simulink model "eCS_Algo_Simulation_2015b"  (R2015b)
settings: Solver=ode1  StartTime=0.0  StopTime=3  FixedStep=1/80000  RelTol=1e-3
PreLoadFcn:
  | if exist('tl_preloadfcn','file'), tl_preloadfcn(gcs,402); end
PostLoadFcn:
  | , if any(exist('dsrtsu_mdlpostloadfcn', 'file') == [2, 3, 6]), try dsrtsu_mdlpostloadfcn('Execute', bdroot); catch fprintf('Error in PostLoadFcn (dsrtsu_mdlpostloadfcn) for model "%s":\n %s\n', bdroot, lasterr); end, end,
  | if exist('tl_postloadfcn','file'), tl_postloadfcn(gcs,402); end
InitFcn:
  | Omegan=1.3024e+03;
  | xi=0.9; %0.48
  | K=0.1931;
  | K1=0.0198;
  | TauLocked=0.00255;
  | TauUnLocked=0.0042;
  | Kp=1/(2*K1);
  | Ki=Kp/((TauLocked+TauUnLocked)/2);
  | if exist('tlds_init','file'), tlds_init(gcs); end
StartFcn:
  | if exist('tlds_start','file'), tlds_start(gcs); end
StopFcn:
  | if exist('tlds_stop','file'), tlds_stop(gcs); end
model workspace (MAT data in the model file):
  au8PrevExecProfile = [0 0 0 0 0 0]
values from neighbouring files (symbols this model uses):
  AccSensor = 5    [Parameter_eCS_Algo.m]
  AlgoType = 0    [Parameter_eCS_Algo.m]
  Cxy = 1*0.017    (= 0.017)    [Acc_Init_SelV1.m]
  Cxz = 1*0.017    (= 0.017)    [Acc_Init_SelV1.m]
  Cyx = 1*0.017    (= 0.017)    [Acc_Init_SelV1.m]
  Cyz = 1*0.017    (= 0.017)    [Acc_Init_SelV1.m]
  Czx = 1*0.017    (= 0.017)    [Acc_Init_SelV1.m]
  Czy = 1*0.017    (= 0.017)    [Acc_Init_SelV1.m]
  Forced_Oscillation = 0    [Parameter_eCS_Algo.m]    (also in run_Rotation_sim.m = run)
  FreqTemperature = 10    [Acc_Init_SelV1.m]
  MaxSensorOffset = 0.3    [Acc_Init_SelV1.m]
  Mean_x_noise = 4e-3    (= 0.004)    [Acc_Init_SelV1.m]
  Mean_y_noise = 4e-3    (= 0.004)    [Acc_Init_SelV1.m]
  Mean_z_noise = 4e-3    (= 0.004)    [Acc_Init_SelV1.m]
  ODR = 8000    [Acc_Init_SelV1.m]
  offsetcorrection_on_off = 0    [Parameter_eCS_Algo.m]
  phi_pulse_rotation = 0    [Parameter_eCS_Algo.m]    (also in run_Rotation_sim.m = angle)
  pulsetype = 2    [Parameter_eCS_Algo.m]    (also in run_simulation.m = j; run_simulation_ActiveX.m = j)
  Range = 4    [Acc_Init_SelV1.m]
  sensitivity_optimisation = 0    [Parameter_eCS_Algo.m]
  TempBias = 0    [Acc_Init_SelV1.m]
  TemperatureAmp = 0    [Acc_Init_SelV1.m]
  Var_x_noise = 1.84e-9    (= 1.84e-09)    [Acc_Init_SelV1.m]
  Var_y_noise = 2.025e-09    [Acc_Init_SelV1.m]
  Var_z_noise = 1.374e-09    [Acc_Init_SelV1.m]
  w_x = 2*pi*F_x    (= 376.991118431)    [Acc_Init_SelV1.m]
  w_y = 2*pi*F_y    (= 376.991118431)    [Acc_Init_SelV1.m]
  w_z = 2*pi*F_z    (= 376.991118431)    [Acc_Init_SelV1.m]
  x_max_temp_drift = 0.061    [Acc_Init_SelV1.m]
  x_offset_enable = 0    [Acc_Init_SelV1.m]
  x_run_to_run_drift = 0.0    (= 0)    [Acc_Init_SelV1.m]
  x_temp_co_drift = 0.000    (= 0)    [Acc_Init_SelV1.m]
  Xi_x = 0.7    [Acc_Init_SelV1.m]
  Xi_y = 0.7    [Acc_Init_SelV1.m]
  Xi_z = 0.7    [Acc_Init_SelV1.m]
  y_max_temp_drift = 0.061    [Acc_Init_SelV1.m]
  y_offset_enable = 0    [Acc_Init_SelV1.m]
  y_run_to_run_drift = 0.0    (= 0)    [Acc_Init_SelV1.m]
  y_temp_co_drift = 0.000    (= 0)    [Acc_Init_SelV1.m]
  z_max_temp_drift = 0.13    [Acc_Init_SelV1.m]
  z_offset_enable = 0    [Acc_Init_SelV1.m]
  z_run_to_run_drift = 0.0    (= 0)    [Acc_Init_SelV1.m]
  z_temp_co_drift = 0.000    (= 0)    [Acc_Init_SelV1.m]
undefined symbols (not defined in the file or in its folder): controller_sample_rate, ddv, DiscIntNeverNeededParam, gmw_roada_x__m_s__, gmw_roada_y__m_s__, gmw_roadtime_2kHz, KSF_50_a_x, KSF_50_a_y, KSF_50_time, KSG_30_a_x, KSG_30_a_y, KSG_30_time, Meldorf_HindenburgstraAcceleration_x__m_s_2_, Meldorf_HindenburgstraAcceleration_y__m_s_2_, Meldorf_HindenburgstraAcceleration_z__m_s_2_, Meldorf_HindenburgstraTime__s_, pulse_FF27, pulse_MPDB, pulse_ODB40, pulse_ODB64, pulse_USNCAP, pulsetime_FF27, pulsetime_MPDB, pulsetime_ODB40, pulsetime_ODB64, pulsetime_USNCAP, Rauasphalt_60_a_x, Rauasphalt_60_a_y, Rauasphalt_60_time, sigbuilder_block, VW_416_2kHza_x_2kHz, VW_416_2kHza_y_2kHz, VW_416_2kHztime_2kHz
libraries: simulink x29, tllib x23, tl_autosar_lib x15, simulink_extras x7, LIB_TF_G_111 x2, LIB_TF_G_12_StepControl x2, LIB_TF_G_112 x1, dspsigops x1
(part 3 of 13)

== system eCS_Algo_Simulation_2015b/µC Signalverarbeitung und Algorithmus2/Calculate Onset >=Threshold/Calculate Onset x-Axis ==
  Acceleration [g] : Inport
  Detect Change : simulink/Logic and Bit Operations/Detect Change  vinit=0  OutDataTypeStr=boolean
  Faktor2 : SampleTimeMath  TsampMathOp=/  TsampMathImp=Offline Scaling Adjustment
  Gain : Gain  Gain=10000/100000
  Triggered Subsystem : Subsystem  TreatAsAtomicUnit=on
  delta x : Sum  Inputs=+-
  Onset [g/s] : Outport
  wires:
  Gain/1 -> Onset [g/s]/1
  Faktor2/1 -> Triggered Subsystem/1(In), Detect Change/1, delta x/1
  Detect Change/1 -> Triggered Subsystem/Trigger
  Triggered Subsystem/1(Out1) -> delta x/2
  delta x/1 -> Gain/1
  Acceleration [g]/1 -> Faktor2/1

== system eCS_Algo_Simulation_2015b/µC Signalverarbeitung und Algorithmus2/Calculate Onset >=Threshold/Calculate Onset y-Axis ==
  Acceleration [g] : Inport
  Detect Change : simulink/Logic and Bit Operations/Detect Change  vinit=0  OutDataTypeStr=boolean
  Faktor2 : SampleTimeMath  TsampMathOp=/  TsampMathImp=Offline Scaling Adjustment
  Gain : Gain  Gain=10000/100000
  Triggered Subsystem : Subsystem  TreatAsAtomicUnit=on
  delta x : Sum  Inputs=+-
  Onset [g/s] : Outport
  wires:
  Acceleration [g]/1 -> Faktor2/1
  delta x/1 -> Gain/1
  Triggered Subsystem/1(Out1) -> delta x/2
  Detect Change/1 -> Triggered Subsystem/Trigger
  Faktor2/1 -> Triggered Subsystem/1(In), delta x/1, Detect Change/1
  Gain/1 -> Onset [g/s]/1

== system eCS_Algo_Simulation_2015b/µC Signalverarbeitung und Algorithmus2/Calculate Onset >=Threshold/Calculate Onset z-Axis ==
  Acceleration [g] : Inport
  Detect Change : simulink/Logic and Bit Operations/Detect Change  vinit=0  OutDataTypeStr=boolean
  Faktor2 : SampleTimeMath  TsampMathOp=/  TsampMathImp=Offline Scaling Adjustment
  Gain : Gain  Gain=10000/100000
  Sample and Hold : dspsigops/Sample and Hold  Commented=on  trig=Rising edge  initCond=-controller_sample_rate  latchinput=on
  Triggered Subsystem : Subsystem  TreatAsAtomicUnit=on
  delta x : Sum  Inputs=+-
  Onset [g/s] : Outport
  wires:
  Gain/1 -> Onset [g/s]/1
  Faktor2/1 -> Triggered Subsystem/1(In), Detect Change/1, delta x/1
  Detect Change/1 -> Triggered Subsystem/Trigger
  Triggered Subsystem/1(Out1) -> delta x/2
  delta x/1 -> Gain/1
  Acceleration [g]/1 -> Faktor2/1

== system eCS_Algo_Simulation_2015b/FSM/Subsystem/FSM/FSM ==
  prrEcsAlgoFlag : Inport
  prrVehicleInputs : Inport  Port=2
  prrExecutedProfiles : Inport  Port=3
  prrLdoAutotestResults : Inport  Port=4
  BusSelector : BusSelector  OutputSignals=b8EcsFlag,u16BallPosition
  BusSelector1 : BusSelector  OutputSignals=u16Vx,u8BuckleState
  BusSelector2 : BusSelector  OutputSignals=u8ExecutedProfile,u8ExecutedProfileOld
  FSM_runCheckVehicleInputs : Subsystem  TreatAsAtomicUnit=on
  FSM_runMainFunction : Subsystem  TreatAsAtomicUnit=on
  PP_psrFsmProfile : tl_autosar_lib/SWC SenderPort  data={'softwarecomponent','AUTOLIV/SoftwareComponents/FSM/FSM','port','psrFsmProfile','date',738308.66468155093}  displaystring=FSM\npsrFsmProfile
  PP_psrSolenoidState : tl_autosar_lib/SWC SenderPort  data={'softwarecomponent','AUTOLIV/SoftwareComponents/FSM/FSM','port','psrSolenoidState','date',738308.6646808217}  displaystring=FSM\npsrSolenoidState
  RP_prrEcsAlgoFlag : tl_autosar_lib/SWC ReceiverPort  data={'softwarecomponent','AUTOLIV/SoftwareComponents/FSM/FSM','port','prrEcsAlgoFlag','date',738304.65103918978}  displaystring=FSM\nprrEcsAlgoFlag
  RP_prrExecutedProfiles : tl_autosar_lib/SWC ReceiverPort  data={'softwarecomponent','AUTOLIV/SoftwareComponents/FSM/FSM','port','prrExecutedProfiles','date',738314.4322294445}  displaystring=FSM\nprrExecutedProfiles
  RP_prrLdoAutotestResults : tl_autosar_lib/SWC ReceiverPort  data={'softwarecomponent','AUTOLIV/SoftwareComponents/FSM/FSM','port','prrLdoAutotestResults','date',738560.69044597226}  displaystring=FSM\nprrLdoAutotestResults
  RP_prrVehicleInputs : tl_autosar_lib/SWC ReceiverPort  data={'softwarecomponent','AUTOLIV/SoftwareComponents/FSM/FSM','port','prrVehicleInputs','date',738304.65103979164}  displaystring=FSM\nprrVehicleInputs
  Terminator{,1..3} (4 alike) : Terminator
  psrSolenoidState : Outport
  psrFsmProfile : Outport  Port=2
  pclPwmServices_SetDutyCycle : Outport  Port=3
  wires:
  prrEcsAlgoFlag/1 -> RP_prrEcsAlgoFlag/1
  RP_prrEcsAlgoFlag/1 -> BusSelector/1
  prrVehicleInputs/1 -> RP_prrVehicleInputs/1
  RP_prrVehicleInputs/1 -> BusSelector1/1
  BusSelector/1 -> FSM_runMainFunction/1(drparg_b8EcsFlag)  "<b8EcsFlag>"
  BusSelector1/1 -> FSM_runCheckVehicleInputs/1(drparg_u16Vx)  "<u16Vx>"
  BusSelector1/2 -> FSM_runCheckVehicleInputs/2(drparg_u8BuckleState)  "<u8BuckleState>"
  FSM_runCheckVehicleInputs/1(ab8IsSolenoidUsed) -> FSM_runMainFunction/2(ab8IsSolenoidUsed)  "ab8IsSolenoidUsed"
  PP_psrSolenoidState/1 -> psrSolenoidState/1
  PP_psrFsmProfile/1 -> psrFsmProfile/1
  FSM_runMainFunction/1(au8FsmState) -> PP_psrSolenoidState/1  "au8SolenoidState"
  FSM_runMainFunction/2(au8SelectedProfile) -> PP_psrFsmProfile/1  "au8SelectedProfile"
  prrExecutedProfiles/1 -> RP_prrExecutedProfiles/1
  RP_prrExecutedProfiles/1 -> BusSelector2/1
  BusSelector2/1 -> FSM_runMainFunction/3(drparg_u8ExecutedProfile)  "<u8ExecutedProfile>"
  BusSelector2/2 -> FSM_runMainFunction/4(drparg_u8ExecutedProfileOld)  "<u8ExecutedProfileOld>"
  FSM_runMainFunction/3(Buck_SetDutyCycle) -> pclPwmServices_SetDutyCycle/1  "pclPwmServices_SetDutyCycle"
  prrLdoAutotestResults/1 -> RP_prrLdoAutotestResults/1
  RP_prrLdoAutotestResults/1 -> FSM_runCheckVehicleInputs/3(drparg_stLdoTestsResults)  "stLdoTestsResults"
  FSM_runMainFunction/6(Buck2_SetDutyCycle) -> Terminator/1
  FSM_runMainFunction/4(EN_Buck) -> Terminator1/1
  BusSelector/2 -> Terminator2/1  "<u16BallPosition>"
  FSM_runMainFunction/5(EN_Buck2) -> Terminator3/1

== system eCS_Algo_Simulation_2015b/SAD/Subsystem/SAD/SAD ==
  prrFsmProfile : Inport
  sim_au16Current : Inport  Port=2
  BusCreator : BusCreator  Inputs=2
  PP_pseSolenoidPWM : tl_autosar_lib/SWC SenderPort  data={'softwarecomponent','AUTOLIV/SoftwareComponents/SAD/SAD','port','pseSolenoidPWM','date',738464.41481978004}  displaystring=SAD\npseSolenoidPWM
  PP_psrExecutedProfiles : tl_autosar_lib/SWC SenderPort  data={'softwarecomponent','AUTOLIV/SoftwareComponents/SAD/SAD','port','psrExecutedProfiles','date',738430.41689956014}  displaystring=SAD\npsrExecutedProfiles
  RP_prrFsmProfile : tl_autosar_lib/SWC ReceiverPort  data={'softwarecomponent','AUTOLIV/SoftwareComponents/SAD/SAD','port','prrFsmProfile','date',738430.41689993057}  displaystring=SAD\nprrFsmProfile
  SAD_Init : Subsystem  TreatAsAtomicUnit=on
  SAD_runMainFunction : Subsystem  TreatAsAtomicUnit=on
  SWC ReceiverPort : tl_autosar_lib/SWC ReceiverPort  data={'softwarecomponent','AUTOLIV/SoftwareComponents/SAD/SAD','port','prrSolenoidCurrent','date',738433.42499521992}  displaystring=SAD\nprrSolenoidCurrent
  SWC SenderPort : tl_autosar_lib/SWC SenderPort  data={'softwarecomponent','AUTOLIV/SoftwareComponents/SAD/SAD','port','sim_psrSolenoidPWM','date',738433.41609917826}  displaystring=SAD\nsim_psrSolenoidPWM
  Terminator : Terminator
  Terminator1 : Terminator
  psrExecutedProfiles : Outport
  sim_au16Pwm : Outport  Port=2
  pseSolenoidPWM : Outport  Port=3
  wires:
  prrFsmProfile/1 -> RP_prrFsmProfile/1
  PP_psrExecutedProfiles/1 -> psrExecutedProfiles/1
  BusCreator/1 -> PP_psrExecutedProfiles/1
  RP_prrFsmProfile/1 -> SAD_runMainFunction/1(drparg_au8SelectedProfile)  "au8SelectedProfile"
  SAD_runMainFunction/1(dsp_u8ExecutedProfile) -> BusCreator/1  "u8ExecutedProfile"
  SAD_runMainFunction/2(dsp_u8ExecutedProfileOld) -> BusCreator/2  "u8ExecutedProfileOld"
  SAD_Init/1(stProfileCfg) -> SAD_runMainFunction/2(stProfileCfg)  "stProfileCfg"
  SAD_runMainFunction/3(sim_au16Pwm) -> SWC SenderPort/1
  SWC SenderPort/1 -> sim_au16Pwm/1
  sim_au16Current/1 -> SWC ReceiverPort/1
  SWC ReceiverPort/1 -> SAD_runMainFunction/3(sim_au16Current)
  PP_pseSolenoidPWM/1 -> pseSolenoidPWM/1
  SAD_runMainFunction/4(dsp_au16Pwm) -> PP_pseSolenoidPWM/1  "au16Pwm"
  SAD_Init/2(EN_Boost_1) -> Terminator/1
  SAD_Init/3(EN_Boost_2) -> Terminator1/1

== system eCS_Algo_Simulation_2015b/eCS/Subsystem/eCS/eCS ==
  prrAccelMtrPerSecSqd : Inport
  prrEcsDiagRequest : Inport  Port=2
  prrSensitivityOpt : Inport  Port=3
  BusCreator : BusCreator  Inputs=2
  PP_psrEcsAlgoData : tl_autosar_lib/SWC SenderPort  data={'softwarecomponent','AUTOLIV/SoftwareComponents/eCS/eCS','port','psrEcsAlgoData','date',738573.71918493055}  displaystring=eCS\npsrEcsAlgoData
  RP_prrAccelMtrPerSecSqd : tl_autosar_lib/SWC ReceiverPort  data={'softwarecomponent','AUTOLIV/SoftwareComponents/eCS/eCS','port','prrAccelMtrPerSecSqd','date',738573.71918538189}  displaystring=eCS\nprrAccelMtrPerSecSqd
  RP_prrEcsDiagRequest : tl_autosar_lib/SWC ReceiverPort  data={'softwarecomponent','AUTOLIV/SoftwareComponents/eCS/eCS','port','prrEcsDiagRequest','date',738573.71918555559}  displaystring=eCS\nprrEcsDiagRequest
  SWC ReceiverPort : tl_autosar_lib/SWC ReceiverPort  data={'softwarecomponent','AUTOLIV/SoftwareComponents/eCS/eCS','port','prrSensitivityOpt','date',738576.35715353012}  displaystring=eCS\nprrSensitivityOpt
  eCS_runMainFunction : Subsystem  TreatAsAtomicUnit=on
  psrEcsAlgoData : Outport
  wires:
  prrAccelMtrPerSecSqd/1 -> RP_prrAccelMtrPerSecSqd/1
  prrEcsDiagRequest/1 -> RP_prrEcsDiagRequest/1
  PP_psrEcsAlgoData/1 -> psrEcsAlgoData/1
  BusCreator/1 -> PP_psrEcsAlgoData/1
  RP_prrAccelMtrPerSecSqd/1 -> eCS_runMainFunction/1(drparg_stAccelMtrPerSecSqd)  "stAccelMtrPerSecSqd"
  RP_prrEcsDiagRequest/1 -> eCS_runMainFunction/2(drparg_b8DiagReq)  "b8DiagReq"
  eCS_runMainFunction/1(dsp_b8EcsFlag) -> BusCreator/1  "b8EcsFlag"
  eCS_runMainFunction/2(dsp_u16BallPosition) -> BusCreator/2  "u16BallPosition"
  prrSensitivityOpt/1 -> SWC ReceiverPort/1
  SWC ReceiverPort/1 -> eCS_runMainFunction/3(drparg_b8IsSensitivityOpt)

== system eCS_Algo_Simulation_2015b/µC Signalverarbeitung und Algorithmus2/Calculate Onset >=Threshold/Calculate Onset x-Axis/Triggered Subsystem ==
  In : Inport  LatchByDelayingOutsideSignal=on
  Trigger : TriggerPort
  Out1 : Outport
  wires:
  In/1 -> Out1/1

== system eCS_Algo_Simulation_2015b/µC Signalverarbeitung und Algorithmus2/Calculate Onset >=Threshold/Calculate Onset y-Axis/Triggered Subsystem ==
  In : Inport  LatchByDelayingOutsideSignal=on
  Trigger : TriggerPort
  Out1 : Outport
  wires:
  In/1 -> Out1/1

== system eCS_Algo_Simulation_2015b/µC Signalverarbeitung und Algorithmus2/Calculate Onset >=Threshold/Calculate Onset z-Axis/Triggered Subsystem ==
  In : Inport  LatchByDelayingOutsideSignal=on
  Trigger : TriggerPort
  Out1 : Outport
  wires:
  In/1 -> Out1/1

== system eCS_Algo_Simulation_2015b/FSM/Subsystem/FSM/FSM/FSM_runCheckVehicleInputs ==
  drparg_u16Vx : Inport  PortDimensions=1  mask(TL_Inport){data={'autosar',{'useautosarcommunication',1,'senderreceiverport','prrVehicleInputs','dataelement','u16Vx'},'date',738304.70202324074}}
      settings: CopyFcn=if exist('tl_reset_reviewflag') == 2, tl_reset_reviewflag(gcbh); end  DeleteFcn=if exist('delete_tlblock','file')==2,delete_tlblock(gcbh);end  NameChangeFcn=if exist('rename_tlblock','file')==2,rename_tlblock(gcbh);end  OpenFcn=if exist('tl_open_blockdlg','file')==2,tl_open_blockdlg(gcbh);else,open_system(gcbh,'parameter');end
      mask Help: eval(['if exist(''tl_online_help'',''file'') == 2, tl_online_help(''Topic'',''TL_Inport''),else, web([''jar:file:///'',matlabroot,''/help/toolbox/simulink/help.jar!/slref/' lower(get_param(gcbh,'Blocktype')) '.html''], ''-helpbrowser''),end'])
      mask Display: plot([0.2 0.35 NaN 0.65 0.8],[0 1 NaN 0 1]);
  drparg_u8BuckleState : Inport  Port=2  PortDimensions=1  mask(TL_Inport){data={'autosar',{'useautosarcommunication',1,'senderreceiverport','prrVehicleInputs','dataelement','u8BuckleState'},'date',738304.7020236227}}
      settings: CopyFcn=if exist('tl_reset_reviewflag') == 2, tl_reset_reviewflag(gcbh); end  DeleteFcn=if exist('delete_tlblock','file')==2,delete_tlblock(gcbh);end  NameChangeFcn=if exist('rename_tlblock','file')==2,rename_tlblock(gcbh);end  OpenFcn=if exist('tl_open_blockdlg','file')==2,tl_open_blockdlg(gcbh);else,open_system(gcbh,'parameter');end
      mask Help: eval(['if exist(''tl_online_help'',''file'') == 2, tl_online_help(''Topic'',''TL_Inport''),else, web([''jar:file:///'',matlabroot,''/help/toolbox/simulink/help.jar!/slref/' lower(get_param(gcbh,'Blocktype')) '.html''], ''-helpbrowser''),end'])
      mask Display: plot([0.2 0.35 NaN 0.65 0.8],[0 1 NaN 0 1]);
  drparg_stLdoTestsResults : Inport  Port=3  mask(TL_BusInport){data={'#autoscaling',5,'#message',5,'#output',5,'#logdata',5,'signals',{{'stLdoTestsResults',{'u8OpenLoadResults';'u8ShortCircuitResults';'u8OverCurrentResults';'u8ThermalShutdownResults';'u8ShortToBatteryResults'}}},'autosar',{'useautosarcommunication',1,'senderreceiverport','prrLdoAutotestResults','dataelement','stLdoTestsResults'},'date',738560.69385527773}}
      settings: CopyFcn=if exist('tl_reset_reviewflag') == 2, tl_reset_reviewflag(gcbh); end  DeleteFcn=if exist('delete_tlblock','file')==2,delete_tlblock(gcbh);end  NameChangeFcn=if exist('rename_tlblock','file')==2,rename_tlblock(gcbh);end  OpenFcn=if exist('tl_open_blockdlg','file')==2,tl_open_blockdlg(gcbh);else,open_system(gcbh,'parameter');end
      mask Help: eval(['if exist(''tl_online_help'',''file'') == 2, tl_online_help(''Topic'',''TL_Inport''),else, web([''jar:file:///'',matlabroot,''/help/toolbox/simulink/help.jar!/slref/' lower(get_param(gcbh,'Blocktype')) '.html''], ''-helpbrowser''),end'])
      mask Display: plot([0.2 0.35 NaN 0.65 0.8],[0 1 NaN 0 1]);
  For Iterator Subsystem : Subsystem  TreatAsAtomicUnit=on
  Runnable : tllib/Function  data={'autosar',{'useautosarspecification',1,'softwarecomponent','AUTOLIV/SoftwareComponents/FSM/FSM','runnable','FSM_runCheckVehicleInputs'},'date',738304.7020226157}  displayString=RUNNABLE
  ab8IsSolenoidUsed : Outport  PortDimensions=6  mask(TL_Outport){data={'autosar',{'useautosarcommunication',1,'kind',3,'interrunnablevariable','ab8IsSolenoidUsed'},'date',738373.3646115741}}
      settings: CopyFcn=if exist('tl_reset_reviewflag') == 2, tl_reset_reviewflag(gcbh); end  DeleteFcn=if exist('delete_tlblock','file')==2,delete_tlblock(gcbh);end  NameChangeFcn=if exist('rename_tlblock','file')==2,rename_tlblock(gcbh);end  OpenFcn=if exist('tl_open_blockdlg','file')==2,tl_open_blockdlg(gcbh);else,open_system(gcbh,'parameter');end
      mask Help: eval(['if exist(''tl_online_help'',''file'') == 2, tl_online_help(''Topic'',''TL_Outport''),else, web([''jar:file:///'',matlabroot,''/help/toolbox/simulink/help.jar!/slref/' lower(get_param(gcbh,'Blocktype')) '.html''], ''-helpbrowser''),end'])
      mask Display: plot([0.2 0.35 NaN 0.65 0.8],[0 1 NaN 0 1]);
  wires:
  drparg_u16Vx/1 -> For Iterator Subsystem/1(u16Vx)
  drparg_u8BuckleState/1 -> For Iterator Subsystem/2(u8BuckleState)
  For Iterator Subsystem/1(ab8SolenoidEnable) -> ab8IsSolenoidUsed/1
  drparg_stLdoTestsResults/1 -> For Iterator Subsystem/3(stLdoTestResult)

== system eCS_Algo_Simulation_2015b/FSM/Subsystem/FSM/FSM/FSM_runMainFunction ==
  note: u8Level
  note: Buck PWM management
  drparg_b8EcsFlag : Inport  PortDimensions=1  mask(TL_Inport){data={'autosar',{'useautosarcommunication',1,'senderreceiverport','prrEcsAlgoFlag','dataelement','b8EcsFlag'},'date',738304.65103487263}}
      settings: CopyFcn=if exist('tl_reset_reviewflag') == 2, tl_reset_reviewflag(gcbh); end  DeleteFcn=if exist('delete_tlblock','file')==2,delete_tlblock(gcbh);end  NameChangeFcn=if exist('rename_tlblock','file')==2,rename_tlblock(gcbh);end  OpenFcn=if exist('tl_open_blockdlg','file')==2,tl_open_blockdlg(gcbh);else,open_system(gcbh,'parameter');end
      mask Help: eval(['if exist(''tl_online_help'',''file'') == 2, tl_online_help(''Topic'',''TL_Inport''),else, web([''jar:file:///'',matlabroot,''/help/toolbox/simulink/help.jar!/slref/' lower(get_param(gcbh,'Blocktype')) '.html''], ''-helpbrowser''),end'])
      mask Display: plot([0.2 0.35 NaN 0.65 0.8],[0 1 NaN 0 1]);
  ab8IsSolenoidUsed : Inport  Port=2  PortDimensions=6  mask(TL_Inport){data={'autosar',{'useautosarcommunication',1,'kind',3,'interrunnablevariable','ab8IsSolenoidUsed'},'date',738307.71878736117}}
      settings: CopyFcn=if exist('tl_reset_reviewflag') == 2, tl_reset_reviewflag(gcbh); end  DeleteFcn=if exist('delete_tlblock','file')==2,delete_tlblock(gcbh);end  NameChangeFcn=if exist('rename_tlblock','file')==2,rename_tlblock(gcbh);end  OpenFcn=if exist('tl_open_blockdlg','file')==2,tl_open_blockdlg(gcbh);else,open_system(gcbh,'parameter');end
      mask Help: eval(['if exist(''tl_online_help'',''file'') == 2, tl_online_help(''Topic'',''TL_Inport''),else, web([''jar:file:///'',matlabroot,''/help/toolbox/simulink/help.jar!/slref/' lower(get_param(gcbh,'Blocktype')) '.html''], ''-helpbrowser''),end'])
      mask Display: plot([0.2 0.35 NaN 0.65 0.8],[0 1 NaN 0 1]);
  drparg_u8ExecutedProfile : Inport  Port=3  PortDimensions=6  mask(TL_Inport){data={'logdata',{'loggingmode',1},'autosar',{'useautosarcommunication',1,'senderreceiverport','prrExecutedProfiles','dataelement','u8ExecutedProfile'},'date',738566.73895473382}}
      settings: CopyFcn=if exist('tl_reset_reviewflag') == 2, tl_reset_reviewflag(gcbh); end  DeleteFcn=if exist('delete_tlblock','file')==2,delete_tlblock(gcbh);end  NameChangeFcn=if exist('rename_tlblock','file')==2,rename_tlblock(gcbh);end  OpenFcn=if exist('tl_open_blockdlg','file')==2,tl_open_blockdlg(gcbh);else,open_system(gcbh,'parameter');end
      mask Help: eval(['if exist(''tl_online_help'',''file'') == 2, tl_online_help(''Topic'',''TL_Inport''),else, web([''jar:file:///'',matlabroot,''/help/toolbox/simulink/help.jar!/slref/' lower(get_param(gcbh,'Blocktype')) '.html''], ''-helpbrowser''),end'])
      mask Display: plot([0.2 0.35 NaN 0.65 0.8],[0 1 NaN 0 1]);
  drparg_u8ExecutedProfileOld : Inport  Port=4  PortDimensions=6  mask(TL_Inport){data={'autosar',{'useautosarcommunication',1,'senderreceiverport','prrExecutedProfiles','dataelement','u8ExecutedProfileOld'},'date',738344.68584724539}}
      settings: CopyFcn=if exist('tl_reset_reviewflag') == 2, tl_reset_reviewflag(gcbh); end  DeleteFcn=if exist('delete_tlblock','file')==2,delete_tlblock(gcbh);end  NameChangeFcn=if exist('rename_tlblock','file')==2,rename_tlblock(gcbh);end  OpenFcn=if exist('tl_open_blockdlg','file')==2,tl_open_blockdlg(gcbh);else,open_system(gcbh,'parameter');end
      mask Help: eval(['if exist(''tl_online_help'',''file'') == 2, tl_online_help(''Topic'',''TL_Inport''),else, web([''jar:file:///'',matlabroot,''/help/toolbox/simulink/help.jar!/slref/' lower(get_param(gcbh,'Blocktype')) '.html''], ''-helpbrowser''),end'])
      mask Display: plot([0.2 0.35 NaN 0.65 0.8],[0 1 NaN 0 1]);
  Bitwise Operator : tllib/Bitwise Operator  logicop=AND  UseBitMask=on  BitMask=bin2dec('00000111')  BitMaskRealWorld=Stored Integer  data={'logdata',{'loggingmode',1},'date',738566.66057049774}
  Buck PWM LuT : Lookup_n-D  NumberOfTableDimensions=1  BreakpointsForDimension1=ddv('FSM/NVP/CFG_au16TempInDeg')  BreakpointsForDimension2=[1:3]  IndexSearchMethod=Linear search  Table=ddv('FSM/NVP/CFG_au16BuckPwm')  ExtrapMethod=Clip  InternalRulePriority=Speed  RndMeth=Simplest  InputSameDT=on  mask(TL_Lookup1D){data={'input',{'variable','FSM/NVP/CFG_au16TempInDeg'},'output',{'type','UInt16'},'table',{'variable','FSM/NVP/CFG_au16BuckPwm'},'date',738597.41315780091}}
      settings: CopyFcn=if exist('tl_reset_reviewflag') == 2, tl_reset_reviewflag(gcbh); end  DeleteFcn=if exist('delete_tlblock','file')==2,delete_tlblock(gcbh);end  NameChangeFcn=if exist('rename_tlblock','file')==2,rename_tlblock(gcbh);end  OpenFcn=if exist('tl_open_blockdlg','file')==2,tl_open_blockdlg(gcbh);else,open_system(gcbh,'parameter');end
      mask Help: eval(['if exist(''tl_online_help'',''file'') == 2, tl_online_help(''Topic'',''TL_Lookup1D''),else, web([''jar:file:///'',matlabroot,''/help/toolbox/simulink/help.jar!/slref/' lower(get_param(gcbh,'Blocktype')) '.html''], ''-helpbrowser''),end'])
      mask Display: plot([-0.1, 1.05, NaN, -0.1, 1.05],[.01, .01, NaN, .99, .99]);
  BusCreator{,1..3} (4 alike) : BusCreator  Inputs=2
  Const : Constant  Value=ddv('PWMIF/Macros/Channels/PWMIF_CH_BUCK_1')  mask(TL_Constant){data={'output',{'variable','PWMIF/Macros/Channels/PWMIF_CH_BUCK_1'},'date',738597.35914218752}}
      settings: CopyFcn=if exist('tl_reset_reviewflag') == 2, tl_reset_reviewflag(gcbh); end  DeleteFcn=if exist('delete_tlblock','file')==2,delete_tlblock(gcbh);end  NameChangeFcn=if exist('rename_tlblock','file')==2,rename_tlblock(gcbh);end  OpenFcn=if exist('tl_open_blockdlg','file')==2,tl_open_blockdlg(gcbh);else,open_system(gcbh,'parameter');end
      mask Help: eval(['if exist(''tl_online_help'',''file'') == 2, tl_online_help(''Topic'',''TL_Constant''),else, web([''jar:file:///'',matlabroot,''/help/toolbox/simulink/help.jar!/slref/' lower(get_param(gcbh,'Blocktype')) '.html''], ''-helpbrowser''),end'])
      mask Display: plot([-0.1, 1.05, NaN, -0.1, 1.05],[.01, .01, NaN, .99, .99]);
  Const1 : Constant  Value=1966  mask(TL_Constant){data={'date',738478.39187206014}}
      settings: CopyFcn=if exist('tl_reset_reviewflag') == 2, tl_reset_reviewflag(gcbh); end  DeleteFcn=if exist('delete_tlblock','file')==2,delete_tlblock(gcbh);end  NameChangeFcn=if exist('rename_tlblock','file')==2,rename_tlblock(gcbh);end  OpenFcn=if exist('tl_open_blockdlg','file')==2,tl_open_blockdlg(gcbh);else,open_system(gcbh,'parameter');end
      mask Help: eval(['if exist(''tl_online_help'',''file'') == 2, tl_online_help(''Topic'',''TL_Constant''),else, web([''jar:file:///'',matlabroot,''/help/toolbox/simulink/help.jar!/slref/' lower(get_param(gcbh,'Blocktype')) '.html''], ''-helpbrowser''),end'])
      mask Display: plot([-0.1, 1.05, NaN, -0.1, 1.05],[.01, .01, NaN, .99, .99]);
  Const3 : Constant  Value=32768  mask(TL_Constant){data={'date',738478.39617783565}}
      settings: CopyFcn=if exist('tl_reset_reviewflag') == 2, tl_reset_reviewflag(gcbh); end  DeleteFcn=if exist('delete_tlblock','file')==2,delete_tlblock(gcbh);end  NameChangeFcn=if exist('rename_tlblock','file')==2,rename_tlblock(gcbh);end  OpenFcn=if exist('tl_open_blockdlg','file')==2,tl_open_blockdlg(gcbh);else,open_system(gcbh,'parameter');end
      mask Help: eval(['if exist(''tl_online_help'',''file'') == 2, tl_online_help(''Topic'',''TL_Constant''),else, web([''jar:file:///'',matlabroot,''/help/toolbox/simulink/help.jar!/slref/' lower(get_param(gcbh,'Blocktype')) '.html''], ''-helpbrowser''),end'])
      mask Display: plot([-0.1, 1.05, NaN, -0.1, 1.05],[.01, .01, NaN, .99, .99]);
  Const4 : Constant  Value=ddv('DIOIF/Macros/Channels/DIOIF_CH_EN_BUCK_1')  mask(TL_Constant){data={'output',{'variable','DIOIF/Macros/Channels/DIOIF_CH_EN_BUCK_1'},'date',738597.35860167828}}
      settings: CopyFcn=if exist('tl_reset_reviewflag') == 2, tl_reset_reviewflag(gcbh); end  DeleteFcn=if exist('delete_tlblock','file')==2,delete_tlblock(gcbh);end  NameChangeFcn=if exist('rename_tlblock','file')==2,rename_tlblock(gcbh);end  OpenFcn=if exist('tl_open_blockdlg','file')==2,tl_open_blockdlg(gcbh);else,open_system(gcbh,'parameter');end
      mask Help: eval(['if exist(''tl_online_help'',''file'') == 2, tl_online_help(''Topic'',''TL_Constant''),else, web([''jar:file:///'',matlabroot,''/help/toolbox/simulink/help.jar!/slref/' lower(get_param(gcbh,'Blocktype')) '.html''], ''-helpbrowser''),end'])
      mask Display: plot([-0.1, 1.05, NaN, -0.1, 1.05],[.01, .01, NaN, .99, .99]);
  Const5 : Constant  Value=ddv('DIOIF/Macros/Channels/DIOIF_CH_EN_BUCK_2')  mask(TL_Constant){data={'output',{'variable','DIOIF/Macros/Channels/DIOIF_CH_EN_BUCK_2'},'date',738597.358925162}}
      settings: CopyFcn=if exist('tl_reset_reviewflag') == 2, tl_reset_reviewflag(gcbh); end  DeleteFcn=if exist('delete_tlblock','file')==2,delete_tlblock(gcbh);end  NameChangeFcn=if exist('rename_tlblock','file')==2,rename_tlblock(gcbh);end  OpenFcn=if exist('tl_open_blockdlg','file')==2,tl_open_blockdlg(gcbh);else,open_system(gcbh,'parameter');end
      mask Help: eval(['if exist(''tl_online_help'',''file'') == 2, tl_online_help(''Topic'',''TL_Constant''),else, web([''jar:file:///'',matlabroot,''/help/toolbox/simulink/help.jar!/slref/' lower(get_param(gcbh,'Blocktype')) '.html''], ''-helpbrowser''),end'])
      mask Display: plot([-0.1, 1.05, NaN, -0.1, 1.05],[.01, .01, NaN, .99, .99]);
  Const6 : Constant  Value=ddv('STD_LOW')  mask(TL_Constant){data={'output',{'variable','STD_LOW'},'date',738566.49000547454}}
      settings: CopyFcn=if exist('tl_reset_reviewflag') == 2, tl_reset_reviewflag(gcbh); end  DeleteFcn=if exist('delete_tlblock','file')==2,delete_tlblock(gcbh);end  NameChangeFcn=if exist('rename_tlblock','file')==2,rename_tlblock(gcbh);end  OpenFcn=if exist('tl_open_blockdlg','file')==2,tl_open_blockdlg(gcbh);else,open_system(gcbh,'parameter');end
      mask Help: eval(['if exist(''tl_online_help'',''file'') == 2, tl_online_help(''Topic'',''TL_Constant''),else, web([''jar:file:///'',matlabroot,''/help/toolbox/simulink/help.jar!/slref/' lower(get_param(gcbh,'Blocktype')) '.html''], ''-helpbrowser''),end'])
      mask Display: plot([-0.1, 1.05, NaN, -0.1, 1.05],[.01, .01, NaN, .99, .99]);
  Const7 : Constant  Value=ddv('DIOIF/Macros/IO_Level/DIOIF_STD_HIGH')  mask(TL_Constant){data={'output',{'variable','DIOIF/Macros/IO_Level/DIOIF_STD_HIGH'},'date',738566.68557425926}}
      settings: CopyFcn=if exist('tl_reset_reviewflag') == 2, tl_reset_reviewflag(gcbh); end  DeleteFcn=if exist('delete_tlblock','file')==2,delete_tlblock(gcbh);end  NameChangeFcn=if exist('rename_tlblock','file')==2,rename_tlblock(gcbh);end  OpenFcn=if exist('tl_open_blockdlg','file')==2,tl_open_blockdlg(gcbh);else,open_system(gcbh,'parameter');end
      mask Help: eval(['if exist(''tl_online_help'',''file'') == 2, tl_online_help(''Topic'',''TL_Constant''),else, web([''jar:file:///'',matlabroot,''/help/toolbox/simulink/help.jar!/slref/' lower(get_param(gcbh,'Blocktype')) '.html''], ''-helpbrowser''),end'])
      mask Display: plot([-0.1, 1.05, NaN, -0.1, 1.05],[.01, .01, NaN, .99, .99]);
  Const8 : Constant  Value=ddv('PWMIF/Macros/Channels/PWMIF_CH_BUCK_2')  mask(TL_Constant){data={'output',{'variable','PWMIF/Macros/Channels/PWMIF_CH_BUCK_2'},'date',738597.35934738431}}
      settings: CopyFcn=if exist('tl_reset_reviewflag') == 2, tl_reset_reviewflag(gcbh); end  DeleteFcn=if exist('delete_tlblock','file')==2,delete_tlblock(gcbh);end  NameChangeFcn=if exist('rename_tlblock','file')==2,rename_tlblock(gcbh);end  OpenFcn=if exist('tl_open_blockdlg','file')==2,tl_open_blockdlg(gcbh);else,open_system(gcbh,'parameter');end
      mask Help: eval(['if exist(''tl_online_help'',''file'') == 2, tl_online_help(''Topic'',''TL_Constant''),else, web([''jar:file:///'',matlabroot,''/help/toolbox/simulink/help.jar!/slref/' lower(get_param(gcbh,'Blocktype')) '.html''], ''-helpbrowser''),end'])
      mask Display: plot([-0.1, 1.05, NaN, -0.1, 1.05],[.01, .01, NaN, .99, .99]);
  Determine Transition : Subsystem  TreatAsAtomicUnit=on
  ExecuteState : Subsystem  TreatAsAtomicUnit=on
  Multiport Switch : MultiPortSwitch  DataPortOrder=Specify indices  Inputs=6  DataPortIndices={1,2,4}  DataPortForDefault=Additional data port  DiagnosticForDefault=None  mask(TL_MultiPortSwitch){data={'output',{'type','UInt16'},'date',738589.71235600696}}
      settings: CopyFcn=if exist('tl_reset_reviewflag') == 2, tl_reset_reviewflag(gcbh); end  DeleteFcn=if exist('delete_tlblock','file')==2,delete_tlblock(gcbh);end  NameChangeFcn=if exist('rename_tlblock','file')==2,rename_tlblock(gcbh);end  OpenFcn=if exist('tl_open_blockdlg','file')==2,tl_open_blockdlg(gcbh);else,open_system(gcbh,'parameter');end
      mask Help: eval(['if exist(''tl_online_help'',''file'') == 2, tl_online_help(''Topic'',''TL_MultiPortSwitch''),else, web([''jar:file:///'',matlabroot,''/help/toolbox/simulink/help.jar!/slref/' lower(get_param(gcbh,'Blocktype')) '.html''], ''-helpbrowser''),end'])
      mask Display: plot([-0.1, 1.05, NaN, -0.1, 1.05],[.01, .01, NaN, .99, .99]);
  Runnable : tllib/Function  data={'autosar',{'useautosarspecification',1,'softwarecomponent','AUTOLIV/SoftwareComponents/FSM/FSM','runnable','FSM_runMainFunction'},'date',738304.65103259264}  displayString=RUNNABLE
  Src : Subsystem
  Switch : Switch  Criteria=u2 ~= 0  mask(TL_Switch){data={'output',{'type','AUTOLIV/DioIf_DataDictionnary/ImplementationDataTypes/u8DioIfLvlType'},'date',738566.48839523143}}
      settings: CopyFcn=if exist('tl_reset_reviewflag') == 2, tl_reset_reviewflag(gcbh); end  DeleteFcn=if exist('delete_tlblock','file')==2,delete_tlblock(gcbh);end  NameChangeFcn=if exist('rename_tlblock','file')==2,rename_tlblock(gcbh);end  OpenFcn=if exist('tl_open_blockdlg','file')==2,tl_open_blockdlg(gcbh);else,open_system(gcbh,'parameter');end
      mask Help: eval(['if exist(''tl_online_help'',''file'') == 2, tl_online_help(''Topic'',''TL_Switch''),else, web([''jar:file:///'',matlabroot,''/help/toolbox/simulink/help.jar!/slref/' lower(get_param(gcbh,'Blocktype')) '.html''], ''-helpbrowser''),end'])
      mask Display: plot([-0.1, 1.05, NaN, -0.1, 1.05],[.01, .01, NaN, .99, .99]);
  old state : UnitDelay  InitialCondition=ddv('FSM/astFsm/Components/au8FsmStatesOld')  SampleTime=-1  mask(TL_UnitDelay){data={'output',{'name','$D','inheritscaling',1},'state',{'variable','FSM/astFsm/Components/au8FsmStatesOld'},'date',738331.66886591434}}
      settings: CopyFcn=if exist('tl_reset_reviewflag') == 2, tl_reset_reviewflag(gcbh); end  DeleteFcn=if exist('delete_tlblock','file')==2,delete_tlblock(gcbh);end  NameChangeFcn=if exist('rename_tlblock','file')==2,rename_tlblock(gcbh);end  OpenFcn=if exist('tl_open_blockdlg','file')==2,tl_open_blockdlg(gcbh);else,open_system(gcbh,'parameter');end
      mask Help: eval(['if exist(''tl_online_help'',''file'') == 2, tl_online_help(''Topic'',''TL_UnitDelay''),else, web([''jar:file:///'',matlabroot,''/help/toolbox/simulink/help.jar!/slref/' lower(get_param(gcbh,'Blocktype')) '.html''], ''-helpbrowser''),end'])
      mask Display: plot([-0.1, 1.05, NaN, -0.1, 1.05],[.01, .01, NaN, .99, .99]);
  scp_getMeasure : Subsystem  TreatAsAtomicUnit=on
  au8FsmState : Outport  PortDimensions=6  mask(TL_Outport){data={'logdata',{'loggingmode',1},'autosar',{'useautosarcommunication',1,'senderreceiverport','psrSolenoidState','dataelement','au8SolenoidState'},'date',738314.63122943288}}
      settings: CopyFcn=if exist('tl_reset_reviewflag') == 2, tl_reset_reviewflag(gcbh); end  DeleteFcn=if exist('delete_tlblock','file')==2,delete_tlblock(gcbh);end  NameChangeFcn=if exist('rename_tlblock','file')==2,rename_tlblock(gcbh);end  OpenFcn=if exist('tl_open_blockdlg','file')==2,tl_open_blockdlg(gcbh);else,open_system(gcbh,'parameter');end
      mask Help: eval(['if exist(''tl_online_help'',''file'') == 2, tl_online_help(''Topic'',''TL_Outport''),else, web([''jar:file:///'',matlabroot,''/help/toolbox/simulink/help.jar!/slref/' lower(get_param(gcbh,'Blocktype')) '.html''], ''-helpbrowser''),end'])
      mask Display: plot([0.2 0.35 NaN 0.65 0.8],[0 1 NaN 0 1]);
  au8SelectedProfile : Outport  Port=2  PortDimensions=6  mask(TL_Outport){data={'logdata',{'loggingmode',1},'autosar',{'useautosarcommunication',1,'senderreceiverport','psrFsmProfile','dataelement','au8SelectedProfile'},'date',738314.63131238427}}
      settings: CopyFcn=if exist('tl_reset_reviewflag') == 2, tl_reset_reviewflag(gcbh); end  DeleteFcn=if exist('delete_tlblock','file')==2,delete_tlblock(gcbh);end  NameChangeFcn=if exist('rename_tlblock','file')==2,rename_tlblock(gcbh);end  OpenFcn=if exist('tl_open_blockdlg','file')==2,tl_open_blockdlg(gcbh);else,open_system(gcbh,'parameter');end
      mask Help: eval(['if exist(''tl_online_help'',''file'') == 2, tl_online_help(''Topic'',''TL_Outport''),else, web([''jar:file:///'',matlabroot,''/help/toolbox/simulink/help.jar!/slref/' lower(get_param(gcbh,'Blocktype')) '.html''], ''-helpbrowser''),end'])
      mask Display: plot([0.2 0.35 NaN 0.65 0.8],[0 1 NaN 0 1]);
  Buck_SetDutyCycle : Outport  Port=3  mask(TL_BusOutport){data={'#autoscaling',2,'#message',2,'#output',2,'#logdata',2,'logdata#2',{'loggingmode',1},'signals',{{'SetDutyCycle',{'cu8ChannelID';'cu16DutyCycle'}}},'autosar',{'useautosarcommunication',1,'kind',4,'clientserverport','pclPwmServices','operation','SetDutyCycle'},'date',738478.39676596061}}
      settings: CopyFcn=if exist('tl_reset_reviewflag') == 2, tl_reset_reviewflag(gcbh); end  DeleteFcn=if exist('delete_tlblock','file')==2,delete_tlblock(gcbh);end  NameChangeFcn=if exist('rename_tlblock','file')==2,rename_tlblock(gcbh);end  OpenFcn=if exist('tl_open_blockdlg','file')==2,tl_open_blockdlg(gcbh);else,open_system(gcbh,'parameter');end
      mask Help: eval(['if exist(''tl_online_help'',''file'') == 2, tl_online_help(''Topic'',''TL_Outport''),else, web([''jar:file:///'',matlabroot,''/help/toolbox/simulink/help.jar!/slref/' lower(get_param(gcbh,'Blocktype')) '.html''], ''-helpbrowser''),end'])
      mask Display: plot([0.2 0.35 NaN 0.65 0.8],[0 1 NaN 0 1]);
  EN_Buck : Outport  Port=4  mask(TL_BusOutport){data={'#autoscaling',2,'#message',2,'#output',2,'#logdata',2,'logdata#2',{'loggingmode',1},'signals',{{'WriteChannel',{'u8ChannelID';'u8Level'}}},'autosar',{'useautosarcommunication',1,'kind',4,'clientserverport','pclDioIfServices','operation','WriteChannel'},'date',738566.6924401389}}
      settings: CopyFcn=if exist('tl_reset_reviewflag') == 2, tl_reset_reviewflag(gcbh); end  DeleteFcn=if exist('delete_tlblock','file')==2,delete_tlblock(gcbh);end  NameChangeFcn=if exist('rename_tlblock','file')==2,rename_tlblock(gcbh);end  OpenFcn=if exist('tl_open_blockdlg','file')==2,tl_open_blockdlg(gcbh);else,open_system(gcbh,'parameter');end
      mask Help: eval(['if exist(''tl_online_help'',''file'') == 2, tl_online_help(''Topic'',''TL_Outport''),else, web([''jar:file:///'',matlabroot,''/help/toolbox/simulink/help.jar!/slref/' lower(get_param(gcbh,'Blocktype')) '.html''], ''-helpbrowser''),end'])
      mask Display: plot([0.2 0.35 NaN 0.65 0.8],[0 1 NaN 0 1]);
  EN_Buck2 : Outport  Port=5  mask(TL_BusOutport){data={'#autoscaling',2,'#message',2,'#output',2,'#logdata',2,'logdata#2',{'loggingmode',1},'signals',{{'WriteChannel',{'u8ChannelID';'u8Level'}}},'autosar',{'useautosarcommunication',1,'kind',4,'clientserverport','pclDioIfServices','operation','WriteChannel'},'date',738566.69658076391}}
      settings: CopyFcn=if exist('tl_reset_reviewflag') == 2, tl_reset_reviewflag(gcbh); end  DeleteFcn=if exist('delete_tlblock','file')==2,delete_tlblock(gcbh);end  NameChangeFcn=if exist('rename_tlblock','file')==2,rename_tlblock(gcbh);end  OpenFcn=if exist('tl_open_blockdlg','file')==2,tl_open_blockdlg(gcbh);else,open_system(gcbh,'parameter');end
      mask Help: eval(['if exist(''tl_online_help'',''file'') == 2, tl_online_help(''Topic'',''TL_Outport''),else, web([''jar:file:///'',matlabroot,''/help/toolbox/simulink/help.jar!/slref/' lower(get_param(gcbh,'Blocktype')) '.html''], ''-helpbrowser''),end'])
      mask Display: plot([0.2 0.35 NaN 0.65 0.8],[0 1 NaN 0 1]);
  Buck2_SetDutyCycle : Outport  Port=6  mask(TL_BusOutport){data={'#autoscaling',2,'#message',2,'#output',2,'#logdata',2,'logdata#2',{'loggingmode',1},'signals',{{'SetDutyCycle',{'cu8ChannelID';'cu16DutyCycle'}}},'autosar',{'useautosarcommunication',1,'kind',4,'clientserverport','pclPwmServices','operation','SetDutyCycle'},'date',738478.39676596061}}
      settings: CopyFcn=if exist('tl_reset_reviewflag') == 2, tl_reset_reviewflag(gcbh); end  DeleteFcn=if exist('delete_tlblock','file')==2,delete_tlblock(gcbh);end  NameChangeFcn=if exist('rename_tlblock','file')==2,rename_tlblock(gcbh);end  OpenFcn=if exist('tl_open_blockdlg','file')==2,tl_open_blockdlg(gcbh);else,open_system(gcbh,'parameter');end
      mask Help: eval(['if exist(''tl_online_help'',''file'') == 2, tl_online_help(''Topic'',''TL_Outport''),else, web([''jar:file:///'',matlabroot,''/help/toolbox/simulink/help.jar!/slref/' lower(get_param(gcbh,'Blocktype')) '.html''], ''-helpbrowser''),end'])
      mask Display: plot([0.2 0.35 NaN 0.65 0.8],[0 1 NaN 0 1]);
  wires:
  drparg_b8EcsFlag/1 -> Determine Transition/1(b8EcsFlag)
  ab8IsSolenoidUsed/1 -> Determine Transition/2(ab8IsSolenoidUsed)
  Determine Transition/1(au8State) -> old state/1, au8FsmState/1, ExecuteState/1(au8States)
  drparg_u8ExecutedProfile/1 -> Determine Transition/3(au8ExecutedProfiles)
  drparg_u8ExecutedProfileOld/1 -> Determine Transition/4(au8ExecutedProfilesOld)
  ExecuteState/1(au8FsmProfiles) -> au8SelectedProfile/1
  old state/1 -> Determine Transition/5(au8OldState)
  Const/1 -> BusCreator/1  "cu8ChannelID"
  BusCreator/1 -> Buck_SetDutyCycle/1  "SetDutyCycle"
  Bitwise Operator/1 -> Multiport Switch/1
  Const4/1 -> BusCreator1/1  "u8ChannelID"
  BusCreator1/1 -> EN_Buck/1  "WriteChannel"
  ExecuteState/2(u8BuckEN) -> Switch/2
  Const5/1 -> BusCreator2/1  "u8ChannelID"
  Switch/1 -> BusCreator2/2, BusCreator1/2  "u8Level"
  BusCreator2/1 -> EN_Buck2/1  "WriteChannel"
  Const6/1 -> Switch/3
  Const7/1 -> Switch/1
  Const8/1 -> BusCreator3/1  "cu8ChannelID"
  Multiport Switch/1 -> BusCreator3/2, BusCreator/2  "cu16DutyCycle"
  BusCreator3/1 -> Buck2_SetDutyCycle/1  "SetDutyCycle"
  Const3/1 -> Multiport Switch/5
  Const1/1 -> Multiport Switch/4, Multiport Switch/2
  Buck PWM LuT/1 -> Multiport Switch/3
  ExecuteState/3(u8Profile) -> Bitwise Operator/1
  Src/1(u8TypeOfMeasure) -> scp_getMeasure/1(u8TypeOfMeasure)
  scp_getMeasure/1(u16Measure) -> Buck PWM LuT/1

== system eCS_Algo_Simulation_2015b/SAD/Subsystem/SAD/SAD/SAD_Init ==
  BusCreator : BusCreator  Inputs=2
  BusCreator1 : BusCreator  Inputs=2
  Constant : Constant  Value=ddv('DIOIF/Macros/IO_Level/DIOIF_STD_HIGH')  mask(TL_Constant){data={'output',{'variable','DIOIF/Macros/IO_Level/DIOIF_STD_HIGH'},'date',738597.36695635412}}
      settings: CopyFcn=if exist('tl_reset_reviewflag') == 2, tl_reset_reviewflag(gcbh); end  DeleteFcn=if exist('delete_tlblock','file')==2,delete_tlblock(gcbh);end  NameChangeFcn=if exist('rename_tlblock','file')==2,rename_tlblock(gcbh);end  OpenFcn=if exist('tl_open_blockdlg','file')==2,tl_open_blockdlg(gcbh);else,open_system(gcbh,'parameter');end
      mask Help: eval(['if exist(''tl_online_help'',''file'') == 2, tl_online_help(''Topic'',''TL_Constant''),else, web([''jar:file:///'',matlabroot,''/help/toolbox/simulink/help.jar!/slref/' lower(get_param(gcbh,'Blocktype')) '.html''], ''-helpbrowser''),end'])
      mask Display: plot([-0.1, 1.05, NaN, -0.1, 1.05],[.01, .01, NaN, .99, .99]);
  Constant1 : Constant  Value=ddv('DIOIF/Macros/Channels/DIOIF_CH_EN_BOOST')  mask(TL_Constant){data={'output',{'variable','DIOIF/Macros/Channels/DIOIF_CH_EN_BOOST'},'date',738597.36719569447}}
      settings: CopyFcn=if exist('tl_reset_reviewflag') == 2, tl_reset_reviewflag(gcbh); end  DeleteFcn=if exist('delete_tlblock','file')==2,delete_tlblock(gcbh);end  NameChangeFcn=if exist('rename_tlblock','file')==2,rename_tlblock(gcbh);end  OpenFcn=if exist('tl_open_blockdlg','file')==2,tl_open_blockdlg(gcbh);else,open_system(gcbh,'parameter');end
      mask Help: eval(['if exist(''tl_online_help'',''file'') == 2, tl_online_help(''Topic'',''TL_Constant''),else, web([''jar:file:///'',matlabroot,''/help/toolbox/simulink/help.jar!/slref/' lower(get_param(gcbh,'Blocktype')) '.html''], ''-helpbrowser''),end'])
      mask Display: plot([-0.1, 1.05, NaN, -0.1, 1.05],[.01, .01, NaN, .99, .99]);
  Constant2 : Constant  Value=ddv('DIOIF/Macros/IO_Level/DIOIF_STD_HIGH')  mask(TL_Constant){data={'output',{'variable','DIOIF/Macros/IO_Level/DIOIF_STD_HIGH'},'date',738597.36695635412}}
      settings: CopyFcn=if exist('tl_reset_reviewflag') == 2, tl_reset_reviewflag(gcbh); end  DeleteFcn=if exist('delete_tlblock','file')==2,delete_tlblock(gcbh);end  NameChangeFcn=if exist('rename_tlblock','file')==2,rename_tlblock(gcbh);end  OpenFcn=if exist('tl_open_blockdlg','file')==2,tl_open_blockdlg(gcbh);else,open_system(gcbh,'parameter');end
      mask Help: eval(['if exist(''tl_online_help'',''file'') == 2, tl_online_help(''Topic'',''TL_Constant''),else, web([''jar:file:///'',matlabroot,''/help/toolbox/simulink/help.jar!/slref/' lower(get_param(gcbh,'Blocktype')) '.html''], ''-helpbrowser''),end'])
      mask Display: plot([-0.1, 1.05, NaN, -0.1, 1.05],[.01, .01, NaN, .99, .99]);
  Constant3 : Constant  Value=ddv('DIOIF/Macros/Channels/DIOIF_CH_EN_BOOST_2')  mask(TL_Constant){data={'output',{'variable','DIOIF/Macros/Channels/DIOIF_CH_EN_BOOST_2'},'date',738597.36739057873}}
      settings: CopyFcn=if exist('tl_reset_reviewflag') == 2, tl_reset_reviewflag(gcbh); end  DeleteFcn=if exist('delete_tlblock','file')==2,delete_tlblock(gcbh);end  NameChangeFcn=if exist('rename_tlblock','file')==2,rename_tlblock(gcbh);end  OpenFcn=if exist('tl_open_blockdlg','file')==2,tl_open_blockdlg(gcbh);else,open_system(gcbh,'parameter');end
      mask Help: eval(['if exist(''tl_online_help'',''file'') == 2, tl_online_help(''Topic'',''TL_Constant''),else, web([''jar:file:///'',matlabroot,''/help/toolbox/simulink/help.jar!/slref/' lower(get_param(gcbh,'Blocktype')) '.html''], ''-helpbrowser''),end'])
      mask Display: plot([-0.1, 1.05, NaN, -0.1, 1.05],[.01, .01, NaN, .99, .99]);
  For : Subsystem  TreatAsAtomicUnit=on
  Runnable : tllib/Function  data={'autosar',{'useautosarspecification',1,'softwarecomponent','AUTOLIV/SoftwareComponents/SAD/SAD','runnable','SAD_Init'},'date',738422.45749591431}  displayString=RUNNABLE
  stProfileCfg : Outport  SampleTime=0.001  mask(TL_BusOutport){data={'#autoscaling',2,'#message',2,'#output',2,'#logdata',2,'signals',{{'stProfileCfg',{'au8FollowingProfile';'au8LastStep'}}},'autosar',{'useautosarcommunication',1,'kind',3,'interrunnablevariable','stProfileCfg'},'date',738430.4169029051}}
      settings: CopyFcn=if exist('tl_reset_reviewflag') == 2, tl_reset_reviewflag(gcbh); end  DeleteFcn=if exist('delete_tlblock','file')==2,delete_tlblock(gcbh);end  NameChangeFcn=if exist('rename_tlblock','file')==2,rename_tlblock(gcbh);end  OpenFcn=if exist('tl_open_blockdlg','file')==2,tl_open_blockdlg(gcbh);else,open_system(gcbh,'parameter');end
      mask Help: eval(['if exist(''tl_online_help'',''file'') == 2, tl_online_help(''Topic'',''TL_Outport''),else, web([''jar:file:///'',matlabroot,''/help/toolbox/simulink/help.jar!/slref/' lower(get_param(gcbh,'Blocktype')) '.html''], ''-helpbrowser''),end'])
      mask Display: plot([0.2 0.35 NaN 0.65 0.8],[0 1 NaN 0 1]);
  EN_Boost_1 : Outport  Port=2  mask(TL_BusOutport){data={'#autoscaling',2,'#message',2,'#output',2,'#logdata',2,'signals',{{'WriteChannel',{'u8ChannelID';'u8Level'}}},'autosar',{'useautosarcommunication',1,'kind',4,'clientserverport','pclDioIfServices','operation','WriteChannel'},'date',738430.41690740746}}
      settings: CopyFcn=if exist('tl_reset_reviewflag') == 2, tl_reset_reviewflag(gcbh); end  DeleteFcn=if exist('delete_tlblock','file')==2,delete_tlblock(gcbh);end  NameChangeFcn=if exist('rename_tlblock','file')==2,rename_tlblock(gcbh);end  OpenFcn=if exist('tl_open_blockdlg','file')==2,tl_open_blockdlg(gcbh);else,open_system(gcbh,'parameter');end
      mask Help: eval(['if exist(''tl_online_help'',''file'') == 2, tl_online_help(''Topic'',''TL_Outport''),else, web([''jar:file:///'',matlabroot,''/help/toolbox/simulink/help.jar!/slref/' lower(get_param(gcbh,'Blocktype')) '.html''], ''-helpbrowser''),end'])
      mask Display: plot([0.2 0.35 NaN 0.65 0.8],[0 1 NaN 0 1]);
  EN_Boost_2 : Outport  Port=3  mask(TL_BusOutport){data={'#autoscaling',2,'#message',2,'#output',2,'#logdata',2,'signals',{{'WriteChannel',{'u8ChannelID';'u8Level'}}},'autosar',{'useautosarcommunication',1,'kind',4,'clientserverport','pclDioIfServices','operation','WriteChannel'},'date',738430.41690740746}}
      settings: CopyFcn=if exist('tl_reset_reviewflag') == 2, tl_reset_reviewflag(gcbh); end  DeleteFcn=if exist('delete_tlblock','file')==2,delete_tlblock(gcbh);end  NameChangeFcn=if exist('rename_tlblock','file')==2,rename_tlblock(gcbh);end  OpenFcn=if exist('tl_open_blockdlg','file')==2,tl_open_blockdlg(gcbh);else,open_system(gcbh,'parameter');end
      mask Help: eval(['if exist(''tl_online_help'',''file'') == 2, tl_online_help(''Topic'',''TL_Outport''),else, web([''jar:file:///'',matlabroot,''/help/toolbox/simulink/help.jar!/slref/' lower(get_param(gcbh,'Blocktype')) '.html''], ''-helpbrowser''),end'])
      mask Display: plot([0.2 0.35 NaN 0.65 0.8],[0 1 NaN 0 1]);
  wires:
  For/1(stProfileCfg) -> stProfileCfg/1
  Constant1/1 -> BusCreator/1  "u8ChannelID"
  Constant/1 -> BusCreator/2  "u8Level"
  BusCreator/1 -> EN_Boost_1/1  "WriteChannel"
  Constant3/1 -> BusCreator1/1  "u8ChannelID"
  Constant2/1 -> BusCreator1/2  "u8Level"
  BusCreator1/1 -> EN_Boost_2/1  "WriteChannel"
